simulink model "Inclined_Plane"  (R2018b)
settings: Solver=VariableStepAuto  StartTime=0.0  StopTime=10  RelTol=1e-3
settings Model: Creator=daiba  LastModifiedBy=daiba

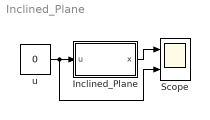
== system Inclined_Plane ==
  Inclined_Plane : Subsystem  mask{m=3, alpha=pi/6, g=9.81, x_zero=0}
      mask prompts: m "Khoi luong vat nang"; alpha "Goc mat phang nghieng"; g "Gia toc trong truong"; x_zero "Vi tri ban dau"
  Scope : Scope  NumInputPorts=2
  u : Constant  Value=0
  wires:
  u/1 -> Scope/2, Inclined_Plane/1(u)
  Inclined_Plane/1(x) -> Scope/1

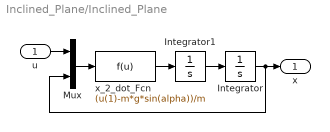
== system Inclined_Plane/Inclined_Plane ==
  u : Inport
  Integrator : Integrator  InitialCondition=x_zero
  Integrator1 : Integrator
  Mux : Mux  Inputs=2
  x_2_dot_Fcn : Fcn  Expr=(u(1)-m*g*sin(alpha))/m
  x : Outport
  wires:
  Mux/1 -> x_2_dot_Fcn/1
  u/1 -> Mux/1
  Integrator/1 -> Mux/2, x/1
  x_2_dot_Fcn/1 -> Integrator1/1
  Integrator1/1 -> Integrator/1
